simulink model "Simulink_rover_Skid_steering_MPC"  (R2013a)
settings: Solver=ode4  StartTime=0.0  StopTime=60  FixedStep=0.06  RelTol=1e-3
model workspace (MAT data in the model file):
  spe_config = []
values from neighbouring files (symbols this model uses):
  M = [Ad Bd;zeros(p,n) eye(p)]    [MPC_Rover_settings.m]
  N = [Bd;eye(p)]    [MPC_Rover_settings.m]    (also in S_Rover_skid_steer.m = 16)
  N1 = 50    [MPC_Rover_settings.m]
  Nu = 10    [MPC_Rover_settings.m]
  Q = [Cd zeros(m,p)]    [MPC_Rover_settings.m]
  Qw = blkdiag(Qw,Qk)    [MPC_Rover_settings.m]
  r = [r;ones(800,1)*pi/2 1*ones(800,1)]    [MPC_Rover_settings.m]    (also in S_Rover_skid_steer.m = 0.2)
  Rw = blkdiag(Rw,Rk)    [MPC_Rover_settings.m]
  Ts = 60e-3    (= 0.06)    [MPC_Rover_settings.m]
settings Model: Creator=obarrero  LastModifiedBy=oscar
settings DataIOCC: SignalLoggingSaveFormat=ModelDataLogs
settings DebuggingCC: UnderspecifiedInitializationDetection=Simplified  MultiTaskDSMMsg=warning  MultiTaskCondExecSysMsg=none  StateNameClashWarn=none  StrictBusMsg=ErrorOnBusTreatedAsVector
settings RTWCC: IncludeERTFirstTime=on
settings GRTTargetCC: CodeReplacementLibrary=None  CPPClassGenCompliant=on

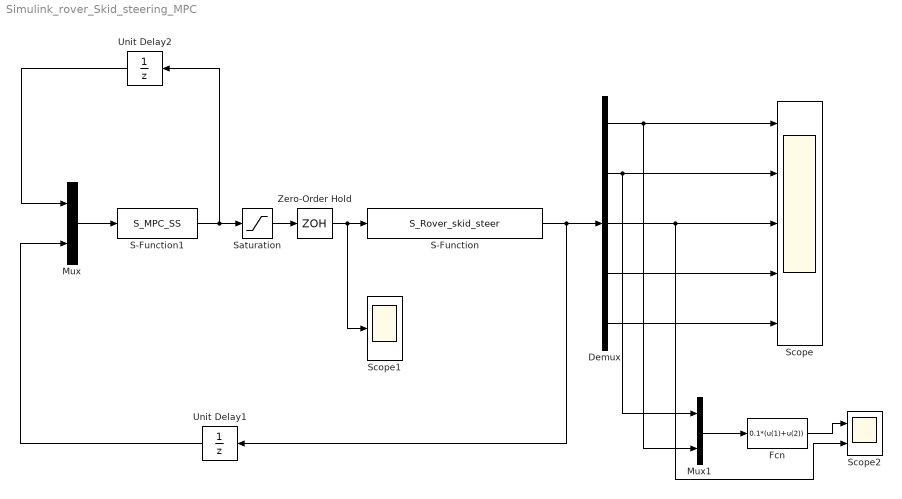
== system Simulink_rover_Skid_steering_MPC ==
  Demux : Demux  Outputs=5
  Fcn : Fcn  Expr=0.1*(u(1)+u(2))  SampleTime=0.06
  Mux : Mux  Inputs=2
  Mux1 : Mux  Inputs=2
  S-Function : S-Function  FunctionName=S_Rover_skid_steer  EnableBusSupport=off
  S-Function1 : S-Function  FunctionName=S_MPC_SS  Parameters=Q,M,N,N1,Nu,Rw,Qw,r  EnableBusSupport=off
  Saturation : Saturate  UpperLimit=100  LowerLimit=-100
  Scope : Scope  NumInputPorts=5
      settings: TimeRange=10  YMin=-1~-0.3~-0.4~-2~1  YMax=1.5~0.9~0.3~5~10
  Scope1 : Scope
      settings: YMin=-1  YMax=1.5
  Scope2 : Scope  NumInputPorts=2
      settings: YMin=-0.1~0.25  YMax=1.1~1.75  SaveName=ScopeData2
  Unit Delay1 : UnitDelay  SampleTime=Ts
  Unit Delay2 : UnitDelay  SampleTime=Ts
  Zero-Order Hold : ZeroOrderHold  SampleTime=0.06
  wires:
  S-Function/1 -> Unit Delay1/1, Demux/1
  Demux/1 -> Mux1/2, Scope/1
  Demux/2 -> Mux1/1, Scope/2
  Demux/3 -> Scope2/2, Scope/3
  Demux/4 -> Scope/4
  Demux/5 -> Scope/5
  Saturation/1 -> Zero-Order Hold/1
  S-Function1/1 -> Unit Delay2/1, Saturation/1
  Mux/1 -> S-Function1/1
  Unit Delay1/1 -> Mux/2
  Unit Delay2/1 -> Mux/1
  Zero-Order Hold/1 -> Scope1/1, S-Function/1
  Mux1/1 -> Fcn/1
  Fcn/1 -> Scope2/1
